simulink model "Zheng_simulation"  (R2018b)
settings: Solver=ode45  StartTime=0.0  StopTime=0.2  RelTol=1e-3  EnableMultiTasking=on
libraries: powerlib x17, powerlib_meascontrol x1
settings Model: Creator=Kumar Pranshu  LastModifiedBy=Hp
settings DataIOCC: LimitDataPoints=on  SaveFormat=Array
settings OptimizationCC: LifeSpan=inf
settings DebuggingCC: SolverPrmCheckMsg=warning  SFUnexpectedBacktrackingDiag=warning  SFNoUnconditionalDefaultTransitionDiag=warning  SFExecutionAtInitializationDiag=none
settings HardwareCC: ProdBitPerPointer=32  ProdBitPerSizeT=32  ProdBitPerPtrDiffT=32  ProdLargestAtomicFloat=None  ProdIntDivRoundTo=Undefined  ProdEndianess=Unspecified  ProdWordSize=32  ProdHWDeviceType=32-bit Generic
settings ModelReferenceCC: PropagateSignalLabelsOutOfModel=off
settings SFSimCC: SimUseLocalCustomCode=off
settings RTWCC: RTWUseLocalCustomCode=off
settings CodeAppCC: StateflowObjectComments=on
settings GRTTargetCC: TargetLangStandard=C89/C90 (ANSI)  GeneratePreprocessorConditionals=Disable all
settings ConfigComp: CovMetricSettings=dw  CovHtmlReporting=on  CovSaveCumulativeToWorkspaceVar=on  CovSaveSingleToWorkspaceVar=on  CovExternalEMLEnable=off  CovSFcnEnable=off
settings SimscapeCC: SimscapeNormalizeSystem=off

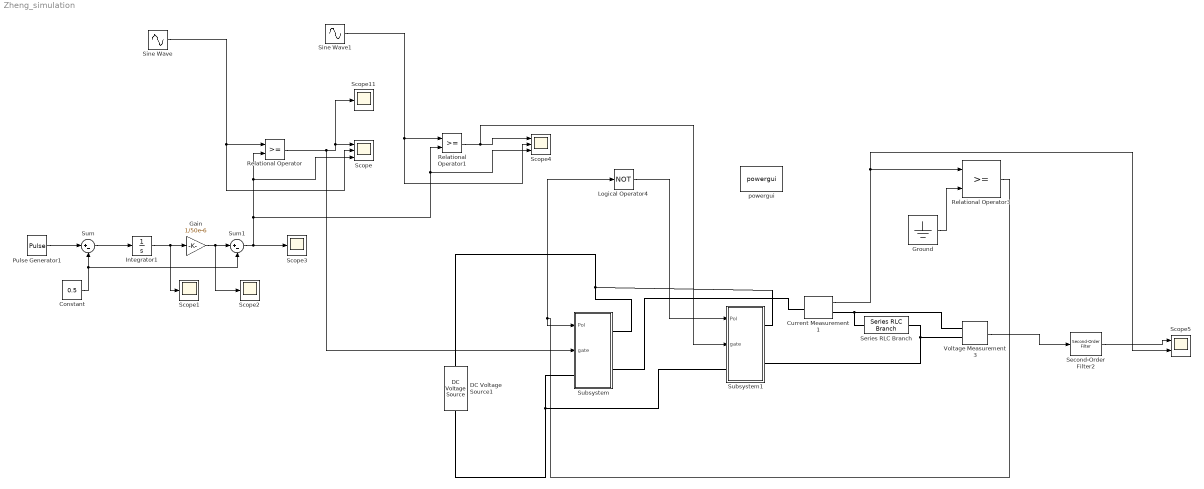
== system Zheng_simulation ==
  Constant : Constant  Value=0.5
  Current Measurement1 : powerlib/Measurements/Current Measurement  PhasorSimulation=off  OutputType=Complex  PSBequivalent=0
      settings: SourceProductName=Simscape Electrical
  DC Voltage Source1 : powerlib/Electrical Sources/DC Voltage Source  Amplitude=330  Measurements=None
      settings: SourceProductName=Simscape Electrical
  Gain : Gain  Gain=1/50e-6
  Ground : Ground
  Integrator1 : Integrator
  Logical Operator4 : Logic  Operator=NOT  Inputs=1  AllPortsSameDT=off  OutDataTypeStr=boolean
  Pulse Generator1 : DiscretePulseGenerator  PulseType=Time based  Period=200e-6  PulseWidth=50
  Relational Operator : RelationalOperator  OutDataTypeStr=boolean  RndMeth=Nearest
  Relational Operator1 : RelationalOperator  OutDataTypeStr=boolean  RndMeth=Nearest
  Relational Operator3 : RelationalOperator  OutDataTypeStr=boolean  RndMeth=Nearest
  Scope : Scope  NumInputPorts=3
  Scope{1..3,11} (4 alike) : Scope
  Scope4 : Scope  NumInputPorts=3
  Scope5 : Scope  NumInputPorts=2
  Second-Order Filter2 : powerlib_meascontrol/Filters/Second-Order Filter  FilterType=Lowpass  Fo=500  Zeta=0.707  Ts=0  Initialize=on  Vac_Init="[0,  0,  500]"  Vdc_Init=0  PlotResponse=off  FreqRange=[0, 500, 1]
      settings: SourceProductName=Simscape Electrical  SourceProductBaseCode=PS
  Series RLC Branch : powerlib/Elements/Series RLC Branch  LConnTagsString=__new0  RConnTagsString=__new0  BranchType=RL  Resistance=25  Inductance=30/(100*3.14)  SetiL0=off  InitialCurrent=0  Capacitance=0  Setx0=off  InitialVoltage=0  Measurements=None
      settings: SourceProductName=Simscape Electrical
  Sine Wave : Sin  Amplitude=0.4  Frequency=2*pi*50  SampleTime=0
  Sine Wave1 : Sin  Amplitude=0.4  Frequency=2*pi*50  Phase=pi  SampleTime=0
  Subsystem : Subsystem
  Subsystem1 : Subsystem
  Sum : Sum  Inputs=|+-
  Sum1 : Sum  Inputs=|+-
  Voltage Measurement3 : powerlib/Measurements/Voltage Measurement  PhasorSimulation=off  OutputType=Complex  PSBequivalent=0
      settings: SourceProductName=Simscape Electrical
  powergui : powerlib/powergui  Priority=1  SimulationMode=Continuous  SampleTime=50e-6  frequency=60  Iterations=50  frequencyindice=0  Pbase=100e6  ErrMax=1e-4  UnitsV=kV  UnitsW=MW  buscounter=0  FunctionMessages=off  echomessages=off  EnableUseOfTLC=off  CurrentSourceSwitches=on  DisableSnubberDevices=off  DisableRonSwitches=off  DisableVfSwitches=off  DisplayEquations=off  SolverType=Tustin  Interpol=off  ExternalGateDelay=off  methode=off  Ts=0  x0status=blocks  SPID=off  SwTol=0  HookPort=off  RestoreLinks=warning  ResistiveCurrentMeasurement=off  Frange=[0:2:500]  Ylog=off  Xlog=on  ShowGrid=off  save=off  variable=ZData  structure=current  ZoomFFT=off  StartTime=0.0  cycles=1  DisplayStyle=1  fundamental=50  FreqAxis=off  MaxFrequency=1000  frequencyindicesteady=1  RmsSteady=1  display=off
  wires:
  Sine Wave/1 -> Scope/2, Relational Operator/1
  Integrator1/1 -> Scope1/1, Gain/1
  Pulse Generator1/1 -> Sum/1
  Sum/1 -> Integrator1/1
  Constant/1 -> Sum1/2, Sum/2
  Gain/1 -> Scope2/1, Sum1/1
  Sine Wave1/1 -> Scope4/2, Relational Operator1/1
  Relational Operator1/1 -> Subsystem1/2(gate), Scope4/1
  Sum1/1 -> Scope3/1, Scope4/3, Relational Operator1/2, Scope/3, Relational Operator/2
  Relational Operator/1 -> Subsystem/2(gate), Scope11/1, Scope/1
  Ground/1 -> Relational Operator3/2
  Current Measurement1/1 -> Scope5/2, Relational Operator3/1
  Relational Operator3/1 -> Logical Operator4/1, Subsystem/1(Pol)
  Logical Operator4/1 -> Subsystem1/1(Pol)
  Voltage Measurement3/1 -> Second-Order Filter2/1
  Second-Order Filter2/1 -> Scope5/1
  connections:
  Subsystem/RConn1 -- DC Voltage Source1/RConn1 -- Subsystem1/RConn1
  Subsystem/LConn1 -- DC Voltage Source1/LConn1 -- Subsystem1/LConn1
  Series RLC Branch/RConn1 -- Subsystem1/RConn2 -- Voltage Measurement3/LConn2
  Current Measurement1/RConn1 -- Voltage Measurement3/LConn1 -- Series RLC Branch/LConn1
  Current Measurement1/LConn1 -- Subsystem/RConn2

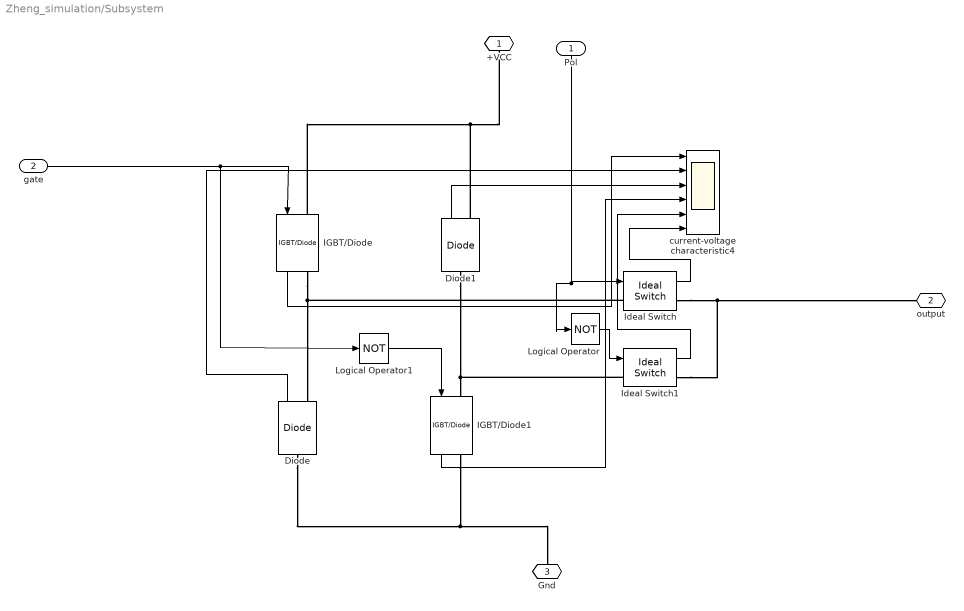
== system Zheng_simulation/Subsystem ==
  Pol : Inport
  gate : Inport  Port=2
  Diode : powerlib/Power Electronics/Diode  Ron=0.001  Lon=0  Vf=0.8  IC=0  UseSnubber=off  Rs=500  Cs=250e-9  Measurements=on
      settings: SourceProductName=Simscape Electrical
  Diode1 : powerlib/Power Electronics/Diode  Ron=0.001  Lon=0  Vf=0.8  IC=0  UseSnubber=off  Rs=500  Cs=250e-9  Measurements=on
      settings: SourceProductName=Simscape Electrical
  IGBT/Diode : powerlib/Power Electronics/IGBT//Diode  Ron=1e-3  Rs=1e5  Cs=inf  Measurements=on
      settings: SourceProductName=Simscape Electrical
  IGBT/Diode1 : powerlib/Power Electronics/IGBT//Diode  Ron=1e-3  Rs=1e5  Cs=inf  Measurements=on
      settings: SourceProductName=Simscape Electrical
  Ideal Switch : powerlib/Power Electronics/Ideal Switch  Ron=0.001  Lon=0  IC=0  Rs=1e7  Cs=inf  Measurements=on
      settings: SourceProductName=Simscape Electrical
  Ideal Switch1 : powerlib/Power Electronics/Ideal Switch  Ron=0.001  Lon=0  IC=0  Rs=1e7  Cs=inf  Measurements=on
      settings: SourceProductName=Simscape Electrical
  Logical Operator : Logic  Operator=NOT  Inputs=1  AllPortsSameDT=off  OutDataTypeStr=boolean
  Logical Operator1 : Logic  Operator=NOT  Inputs=1  AllPortsSameDT=off  OutDataTypeStr=boolean
  current-voltage characteristic4 : Scope  NumInputPorts=6
  +VCC : PMIOPort  Side=Right
  "output " : PMIOPort  Port=2  Side=Right
  Gnd : PMIOPort  Port=3  Side=Left
  wires:
  Ideal Switch/1 -> current-voltage characteristic4/6
  Diode/1 -> current-voltage characteristic4/2
  IGBT/Diode/1 -> current-voltage characteristic4/1
  gate/1 -> Logical Operator1/1, IGBT/Diode/1
  Logical Operator/1 -> Ideal Switch1/1
  Ideal Switch1/1 -> current-voltage characteristic4/5
  Logical Operator1/1 -> IGBT/Diode1/1
  IGBT/Diode1/1 -> current-voltage characteristic4/4
  Diode1/1 -> current-voltage characteristic4/3
  Pol/1 -> Ideal Switch/1, Logical Operator/1
  connections:
  Diode1/LConn1 -- Ideal Switch1/LConn1 -- IGBT/Diode1/LConn1
  IGBT/Diode/RConn1 -- Ideal Switch/LConn1 -- Diode/RConn1
  IGBT/Diode/LConn1 -- +VCC/RConn1 -- Diode1/RConn1
  Diode/LConn1 -- Gnd/RConn1 -- IGBT/Diode1/RConn1
  Ideal Switch/RConn1 -- "output "/RConn1 -- Ideal Switch1/RConn1

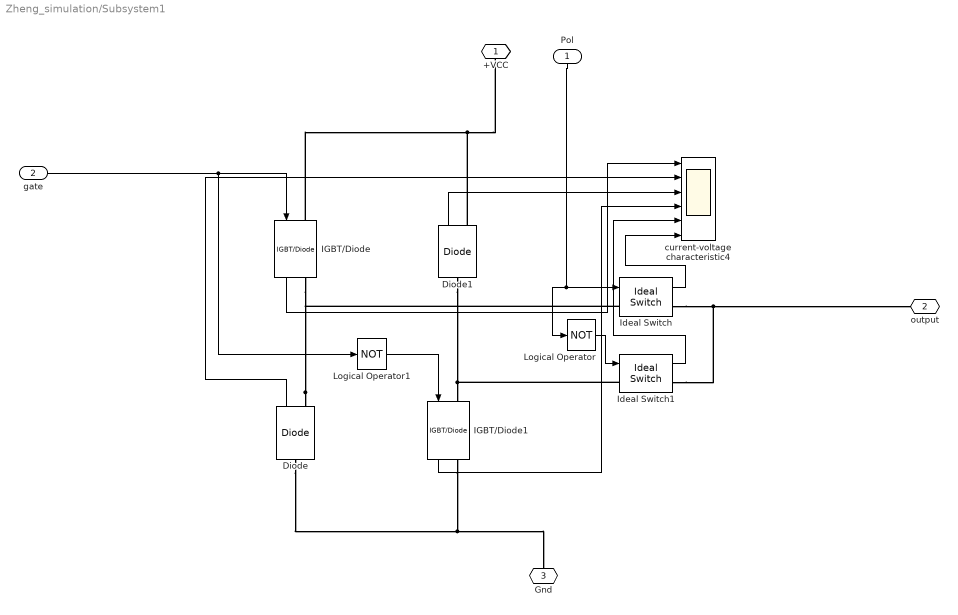
== system Zheng_simulation/Subsystem1 ==
  Pol : Inport
  gate : Inport  Port=2
  Diode : powerlib/Power Electronics/Diode  Ron=0.001  Lon=0  Vf=0.8  IC=0  UseSnubber=off  Rs=500  Cs=250e-9  Measurements=on
      settings: SourceProductName=Simscape Electrical
  Diode1 : powerlib/Power Electronics/Diode  Ron=0.001  Lon=0  Vf=0.8  IC=0  UseSnubber=off  Rs=500  Cs=250e-9  Measurements=on
      settings: SourceProductName=Simscape Electrical
  IGBT/Diode : powerlib/Power Electronics/IGBT//Diode  Ron=1e-3  Rs=1e5  Cs=inf  Measurements=on
      settings: SourceProductName=Simscape Electrical
  IGBT/Diode1 : powerlib/Power Electronics/IGBT//Diode  Ron=1e-3  Rs=1e5  Cs=inf  Measurements=on
      settings: SourceProductName=Simscape Electrical
  Ideal Switch : powerlib/Power Electronics/Ideal Switch  Ron=0.001  Lon=0  IC=0  Rs=1e5  Cs=inf  Measurements=on
      settings: SourceProductName=Simscape Electrical
  Ideal Switch1 : powerlib/Power Electronics/Ideal Switch  Ron=0.001  Lon=0  IC=0  Rs=1e5  Cs=inf  Measurements=on
      settings: SourceProductName=Simscape Electrical
  Logical Operator : Logic  Operator=NOT  Inputs=1  AllPortsSameDT=off  OutDataTypeStr=boolean
  Logical Operator1 : Logic  Operator=NOT  Inputs=1  AllPortsSameDT=off  OutDataTypeStr=boolean
  current-voltage characteristic4 : Scope  NumInputPorts=6
  +VCC : PMIOPort  Side=Right
  "output " : PMIOPort  Port=2  Side=Right
  Gnd : PMIOPort  Port=3  Side=Left
  wires:
  Ideal Switch/1 -> current-voltage characteristic4/6
  Diode/1 -> current-voltage characteristic4/2
  IGBT/Diode/1 -> current-voltage characteristic4/1
  gate/1 -> Logical Operator1/1, IGBT/Diode/1
  Logical Operator/1 -> Ideal Switch1/1
  Ideal Switch1/1 -> current-voltage characteristic4/5
  Logical Operator1/1 -> IGBT/Diode1/1
  IGBT/Diode1/1 -> current-voltage characteristic4/4
  Diode1/1 -> current-voltage characteristic4/3
  Pol/1 -> Ideal Switch/1, Logical Operator/1
  connections:
  Diode1/LConn1 -- IGBT/Diode1/LConn1 -- Ideal Switch1/LConn1
  Diode/RConn1 -- IGBT/Diode/RConn1 -- Ideal Switch/LConn1
  Diode1/RConn1 -- IGBT/Diode/LConn1 -- +VCC/RConn1
  IGBT/Diode1/RConn1 -- Diode/LConn1 -- Gnd/RConn1
  Ideal Switch1/RConn1 -- Ideal Switch/RConn1 -- "output "/RConn1
